simulink model "dout_eml"  (R2014a)
settings: Solver=FixedStepDiscrete  SolverMode=SingleTasking  StartTime=0.0  StopTime=10.0  RelTol=1e-3
settings Model: ExtModeTrigDuration=2  Creator=gcampa  LastModifiedBy=gcampa
settings OptimizationCC: OptimizeModelRefInitCode=on  LifeSpan=1
settings DebuggingCC: UnderspecifiedInitializationDetection=Classic  SolverPrmCheckMsg=none  FrameProcessingCompatibilityMsg=error  StateNameClashWarn=warning
settings HardwareCC: ProdBitPerInt=16  ProdBitPerPointer=8  ProdIntDivRoundTo=Zero  ProdEndianess=LittleEndian  ProdWordSize=8  ProdHWDeviceType=Atmel->AVR
settings RTWCC: SystemTargetFile=realtime.tlc  GenerateMakefile=off  TemplateMakefile=realtime.tmf  Description=Run on Target Hardware  RTWVerbose=off  ProcessScript=realtime_make_rtw_hook  CustomSource=..\src\digitalio_arduino.cpp
settings STFCustomTargetCC: TargetLibSuffix=.a  GenerateSampleERTMain=on  ConcurrentExecutionCompliant=off  GeneratePreprocessorConditionals=Use local settings  ERTCustomFileBanners=on  SupportNonInlinedSFcns=off  SupportVariableSizeSignals=on  MATLABClassNameForMDSCustomization=Simulink.SoftwareTarget.ERTCustomization  GRTInterface=off  SystemTargetFile=realtime.tlc
settings ERTTargetCC: CombineOutputUpdateFcns=off  SupportContinuousTime=on  SupportVariableSizeSignals=on  ExtModeTransport=3  ExtModeMexFile=ext_serial_win32_comm  ExtModeMexArgs=0 1 9600  ERTSrcFileBannerTemplate=realtime_code_template.cgt  ERTHdrFileBannerTemplate=realtime_code_template.cgt  ERTDataSrcFileTemplate=realtime_code_template.cgt  ERTDataHdrFileTemplate=realtime_code_template.cgt  ERTCustomFileTemplate=realtime_file_process.tlc

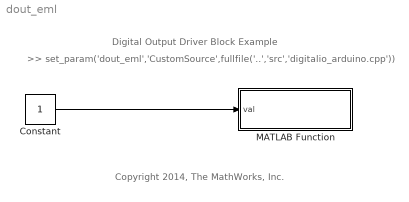
== system dout_eml ==
  note: >> set_param('dout_eml','CustomSource',fullfile('..','src','digitalio_arduino.cpp'))
  note: Digital Output Driver Block Example
  note: Copyright 2014, The MathWorks, Inc.
  Constant : Constant  SampleTime=0.2
  MATLAB Function : MATLAB Function  TreatAsAtomicUnit=on  mask(Digital Write){pin=3, T=0.05}
      mask prompts: T "Sample Time"
      mask help:
      | Every time this block is executed it gets the value (0 or 1) at its input and writes it (as a digital output) to a given pin.
      |
      | The first parameter is the number of the pin where the digital output needs to be performed. The second parameter is the sample time.
      |
      | Note that if this block gets copied to a new model, then the file "digitalio_arduino.cpp" must be added to the CustomSource field of the new model using the "set_param" instruction. See the guide for more info.
  wires:
  Constant/1 -> MATLAB Function/1(val)

== matlab function dout_eml/MATLAB Function ==
  settings: updateMethod=DISCRETE  sampleTime=T
  data: pin parameter; val input
function digitalWrite(pin,val)
%#codegen

persistent initflag;

if strcmp(coder.target, 'rtw'),
    
    if isempty(initflag),
        % Initialize step
        coder.ceval('digitalIOSetup',uint8(pin),true);
        initflag = 1;
    else
        % output Step
        coder.ceval('writeDigitalPin',uint8(pin),logical(val));
    end
    
end
